simulink model "tiaoshi"  (R2014b)
settings: Solver=ode45  StartTime=0.0  StopTime=10.0  RelTol=1e-3
libraries: simulink x4, fuzblock x1
settings Model: Creator=Administrator  LastModifiedBy=Administrator

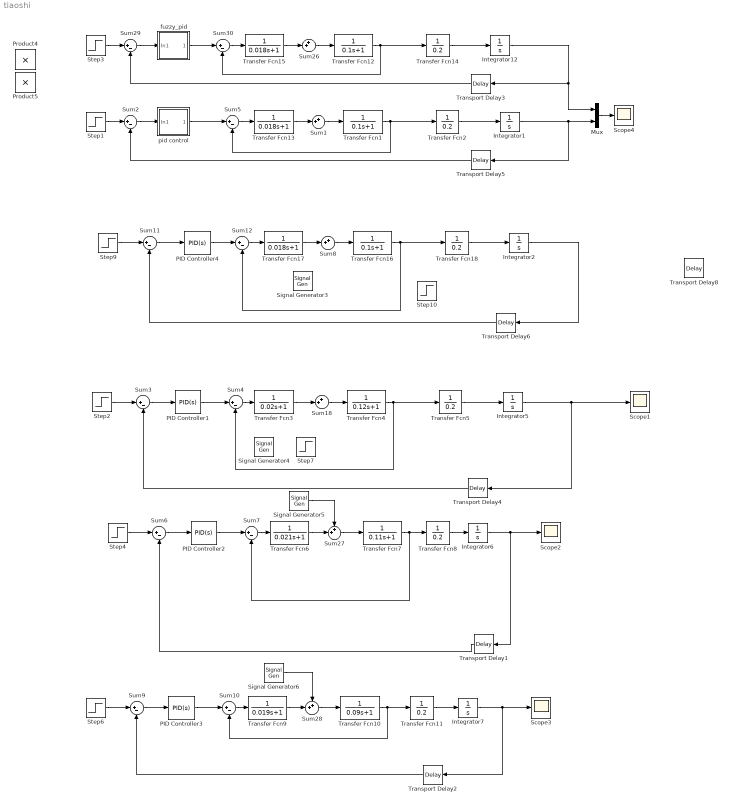
== system tiaoshi ==
  Integrator{1..2,5..7,12} (6 alike) : Integrator
  Mux : Mux  Inputs=2
  PID Controller1 : simulink/Continuous/PID Controller  Controller=PID  TimeDomain=Continuous-time  SampleTime=-1  IntegratorMethod=Forward Euler  FilterMethod=Forward Euler  Form=Parallel  P=4.34348893595362  I=0.409606906541511  D=0.190106280421876  N=113.521570556965  InitialConditionSource=internal  InitialConditionForIntegrator=0  InitialConditionForFilter=0  ExternalReset=none  LimitOutput=off  UpperSaturationLimit=inf  LowerSaturationLimit=-inf  LinearizeAsGain=on  AntiWindupMode=none  Kb=1  TrackingMode=off  Kt=1  PParamMin=[]  PParamMax=[]  IParamMin=[]  IParamMax=[]  DParamMin=[]  DParamMax=[]  NParamMin=[]  NParamMax=[]  KbParamMin=[]  KbParamMax=[]  KtParamMin=[]  KtParamMax=[]  POutMin=[]  POutMax=[]  IOutMin=[]  IOutMax=[]  DOutMin=[]  DOutMax=[]  NOutMin=[]  NOutMax=[]  KbOutMin=[]  KbOutMax=[]  KtOutMin=[]  KtOutMax=[]  IntegratorOutMin=[]  IntegratorOutMax=[]  FilterOutMin=[]  FilterOutMax=[]  SumOutMin=[]  SumOutMax=[]  SumI1OutMin=[]  SumI1OutMax=[]  SumI2OutMin=[]  SumI2OutMax=[]  SumI3OutMin=[]  SumI3OutMax=[]  SumDOutMin=[]  SumDOutMax=[]  SaturationOutMin=[]  SaturationOutMax=[]  IntegratorContinuousStateAttributes=''  IntegratorStateMustResolveToSignalObject=off  IntegratorRTWStateStorageClass=Auto  FilterContinuousStateAttributes=''  FilterStateMustResolveToSignalObject=off  FilterRTWStateStorageClass=Auto  DifferentiatorICPrevScaledInput=0  DifferentiatorOutMin=[]  DifferentiatorOutMax=[]  UseFilter=on
  PID Controller2 : simulink/Continuous/PID Controller  Controller=PID  TimeDomain=Continuous-time  SampleTime=-1  IntegratorMethod=Forward Euler  FilterMethod=Forward Euler  Form=Parallel  P=4.3714761921553  I=0.418612157121434  D=0.176716531069936  N=115.244644738995  InitialConditionSource=internal  InitialConditionForIntegrator=0  InitialConditionForFilter=0  ExternalReset=none  LimitOutput=off  UpperSaturationLimit=inf  LowerSaturationLimit=-inf  LinearizeAsGain=on  AntiWindupMode=none  Kb=1  TrackingMode=off  Kt=1  PParamMin=[]  PParamMax=[]  IParamMin=[]  IParamMax=[]  DParamMin=[]  DParamMax=[]  NParamMin=[]  NParamMax=[]  KbParamMin=[]  KbParamMax=[]  KtParamMin=[]  KtParamMax=[]  POutMin=[]  POutMax=[]  IOutMin=[]  IOutMax=[]  DOutMin=[]  DOutMax=[]  NOutMin=[]  NOutMax=[]  KbOutMin=[]  KbOutMax=[]  KtOutMin=[]  KtOutMax=[]  IntegratorOutMin=[]  IntegratorOutMax=[]  FilterOutMin=[]  FilterOutMax=[]  SumOutMin=[]  SumOutMax=[]  SumI1OutMin=[]  SumI1OutMax=[]  SumI2OutMin=[]  SumI2OutMax=[]  SumI3OutMin=[]  SumI3OutMax=[]  SumDOutMin=[]  SumDOutMax=[]  SaturationOutMin=[]  SaturationOutMax=[]  IntegratorContinuousStateAttributes=''  IntegratorStateMustResolveToSignalObject=off  IntegratorRTWStateStorageClass=Auto  FilterContinuousStateAttributes=''  FilterStateMustResolveToSignalObject=off  FilterRTWStateStorageClass=Auto  DifferentiatorICPrevScaledInput=0  DifferentiatorOutMin=[]  DifferentiatorOutMax=[]  UseFilter=on
  PID Controller3 : simulink/Continuous/PID Controller  Controller=PID  TimeDomain=Continuous-time  SampleTime=-1  IntegratorMethod=Forward Euler  FilterMethod=Forward Euler  Form=Parallel  P=4.54060551459518  I=0.450019772467081  D=0.137661903224342  N=119.172045893014  InitialConditionSource=internal  InitialConditionForIntegrator=0  InitialConditionForFilter=0  ExternalReset=none  LimitOutput=off  UpperSaturationLimit=inf  LowerSaturationLimit=-inf  LinearizeAsGain=on  AntiWindupMode=none  Kb=1  TrackingMode=off  Kt=1  PParamMin=[]  PParamMax=[]  IParamMin=[]  IParamMax=[]  DParamMin=[]  DParamMax=[]  NParamMin=[]  NParamMax=[]  KbParamMin=[]  KbParamMax=[]  KtParamMin=[]  KtParamMax=[]  POutMin=[]  POutMax=[]  IOutMin=[]  IOutMax=[]  DOutMin=[]  DOutMax=[]  NOutMin=[]  NOutMax=[]  KbOutMin=[]  KbOutMax=[]  KtOutMin=[]  KtOutMax=[]  IntegratorOutMin=[]  IntegratorOutMax=[]  FilterOutMin=[]  FilterOutMax=[]  SumOutMin=[]  SumOutMax=[]  SumI1OutMin=[]  SumI1OutMax=[]  SumI2OutMin=[]  SumI2OutMax=[]  SumI3OutMin=[]  SumI3OutMax=[]  SumDOutMin=[]  SumDOutMax=[]  SaturationOutMin=[]  SaturationOutMax=[]  IntegratorContinuousStateAttributes=''  IntegratorStateMustResolveToSignalObject=off  IntegratorRTWStateStorageClass=Auto  FilterContinuousStateAttributes=''  FilterStateMustResolveToSignalObject=off  FilterRTWStateStorageClass=Auto  DifferentiatorICPrevScaledInput=0  DifferentiatorOutMin=[]  DifferentiatorOutMax=[]  UseFilter=on
  PID Controller4 : simulink/Continuous/PID Controller  Controller=PID  TimeDomain=Continuous-time  SampleTime=-1  IntegratorMethod=Forward Euler  FilterMethod=Forward Euler  Form=Parallel  P=7.09807299066698  I=1.09867748930147  D=0.315560684469702  N=2035.68968381362  InitialConditionSource=internal  InitialConditionForIntegrator=0  InitialConditionForFilter=0  ExternalReset=none  LimitOutput=off  UpperSaturationLimit=inf  LowerSaturationLimit=-inf  LinearizeAsGain=on  AntiWindupMode=none  Kb=1  TrackingMode=off  Kt=1  PParamMin=[]  PParamMax=[]  IParamMin=[]  IParamMax=[]  DParamMin=[]  DParamMax=[]  NParamMin=[]  NParamMax=[]  KbParamMin=[]  KbParamMax=[]  KtParamMin=[]  KtParamMax=[]  POutMin=[]  POutMax=[]  IOutMin=[]  IOutMax=[]  DOutMin=[]  DOutMax=[]  NOutMin=[]  NOutMax=[]  KbOutMin=[]  KbOutMax=[]  KtOutMin=[]  KtOutMax=[]  IntegratorOutMin=[]  IntegratorOutMax=[]  FilterOutMin=[]  FilterOutMax=[]  SumOutMin=[]  SumOutMax=[]  SumI1OutMin=[]  SumI1OutMax=[]  SumI2OutMin=[]  SumI2OutMax=[]  SumI3OutMin=[]  SumI3OutMax=[]  SumDOutMin=[]  SumDOutMax=[]  SaturationOutMin=[]  SaturationOutMax=[]  IntegratorContinuousStateAttributes=''  IntegratorStateMustResolveToSignalObject=off  IntegratorRTWStateStorageClass=Auto  FilterContinuousStateAttributes=''  FilterStateMustResolveToSignalObject=off  FilterRTWStateStorageClass=Auto  DifferentiatorICPrevScaledInput=0  DifferentiatorOutMin=[]  DifferentiatorOutMax=[]  UseFilter=on
  Product4 : Product  RndMeth=Zero
  Product5 : Product  RndMeth=Zero
  Scope{1..4} (4 alike) : Scope
      Scope1 settings: SaveName=dianji2
      Scope2 settings: SaveName=dianji3
      Scope3 settings: SaveName=dianji4
      Scope4 settings: SaveName=dianjix
  Signal Generator{3..6} (4 alike) : SignalGenerator  WaveForm=random  Amplitude=10  Frequency=2
  Step{1..3,9} (4 alike) : Step  After=50  SampleTime=0
  Step10 : Step  Time=5  After=-1  SampleTime=0
  Step4 : Step  SampleTime=0
  Step6 : Step  SampleTime=0
  Step7 : Step  Time=5  After=-1  SampleTime=0
  Sum{1,8,18,26..28} (6 alike) : Sum  Inputs=++|
  Sum{2..7,9..12,29..30} (12 alike) : Sum  Inputs=|+-
  Transfer Fcn1 : TransferFcn  Denominator=[0.1 1]
  Transfer Fcn10 : TransferFcn  Denominator=[0.09 1]
  Transfer Fcn{2,5,8,11,14,18} (6 alike) : TransferFcn  Denominator=[0.2]
  Transfer Fcn12 : TransferFcn  Denominator=[0.1 1]
  Transfer Fcn13 : TransferFcn  Denominator=[0.018 1]
  Transfer Fcn15 : TransferFcn  Denominator=[0.018 1]
  Transfer Fcn16 : TransferFcn  Denominator=[0.1 1]
  Transfer Fcn17 : TransferFcn  Denominator=[0.018 1]
  Transfer Fcn3 : TransferFcn  Denominator=[0.02 1]
  Transfer Fcn4 : TransferFcn  Denominator=[0.12 1]
  Transfer Fcn6 : TransferFcn  Denominator=[0.021 1]
  Transfer Fcn7 : TransferFcn  Denominator=[0.11 1]
  Transfer Fcn9 : TransferFcn  Denominator=[0.019 1]
  Transport Delay1 : TransportDelay  DelayTime=0.02
  Transport Delay2 : TransportDelay  DelayTime=0.02
  Transport Delay{3,5..6,8} (4 alike) : TransportDelay  DelayTime=0.004
  Transport Delay4 : TransportDelay  DelayTime=0.02
  fuzzy_pid : Subsystem
  pid control : Subsystem
  wires:
  Step2/1 -> Sum3/1
  Sum3/1 -> PID Controller1/1
  Transfer Fcn4/1 -> Sum4/2, Transfer Fcn5/1
  Sum4/1 -> Transfer Fcn3/1
  PID Controller1/1 -> Sum4/1
  Transfer Fcn5/1 -> Integrator5/1
  Step4/1 -> Sum6/1
  Sum6/1 -> PID Controller2/1
  Transfer Fcn7/1 -> Transfer Fcn8/1, Sum7/2
  Sum7/1 -> Transfer Fcn6/1
  PID Controller2/1 -> Sum7/1
  Transfer Fcn8/1 -> Integrator6/1
  Step6/1 -> Sum9/1
  Sum9/1 -> PID Controller3/1
  Transfer Fcn10/1 -> Transfer Fcn11/1, Sum10/2
  Sum10/1 -> Transfer Fcn9/1
  PID Controller3/1 -> Sum10/1
  Transfer Fcn11/1 -> Integrator7/1
  Integrator6/1 -> Scope2/1, Transport Delay1/1
  Integrator7/1 -> Transport Delay2/1, Scope3/1
  Transfer Fcn3/1 -> Sum18/2
  Sum18/1 -> Transfer Fcn4/1
  Integrator5/1 -> Scope1/1, Transport Delay4/1
  Transport Delay4/1 -> Sum3/2
  Transport Delay1/1 -> Sum6/2
  Transport Delay2/1 -> Sum9/2
  Signal Generator5/1 -> Sum27/1
  Transfer Fcn6/1 -> Sum27/2
  Sum27/1 -> Transfer Fcn7/1
  Transfer Fcn9/1 -> Sum28/2
  Sum28/1 -> Transfer Fcn10/1
  Signal Generator6/1 -> Sum28/1
  Step3/1 -> Sum29/1
  Sum29/1 -> fuzzy_pid/1(In1)
  Transfer Fcn12/1 -> Sum30/2, Transfer Fcn14/1
  Sum30/1 -> Transfer Fcn15/1
  Transfer Fcn14/1 -> Integrator12/1
  Sum26/1 -> Transfer Fcn12/1
  Integrator12/1 -> Mux/1, Transport Delay3/1
  Transport Delay3/1 -> Sum29/2
  Transfer Fcn15/1 -> Sum26/2
  fuzzy_pid/1(Out1) -> Sum30/1
  Step1/1 -> Sum2/1
  Transfer Fcn1/1 -> Sum5/2, Transfer Fcn2/1
  Sum5/1 -> Transfer Fcn13/1
  Transfer Fcn2/1 -> Integrator1/1
  Sum1/1 -> Transfer Fcn1/1
  Integrator1/1 -> Mux/2, Transport Delay5/1
  Transport Delay5/1 -> Sum2/2
  Transfer Fcn13/1 -> Sum1/2
  pid control/1(Out1) -> Sum5/1
  Mux/1 -> Scope4/1
  Step9/1 -> Sum11/1
  Sum11/1 -> PID Controller4/1
  Transfer Fcn16/1 -> Sum12/2, Transfer Fcn18/1
  Sum12/1 -> Transfer Fcn17/1
  Transfer Fcn18/1 -> Integrator2/1
  Sum8/1 -> Transfer Fcn16/1
  Integrator2/1 -> Transport Delay6/1
  Transport Delay6/1 -> Sum11/2
  Transfer Fcn17/1 -> Sum8/2
  PID Controller4/1 -> Sum12/1
  Sum2/1 -> pid control/1(In1)

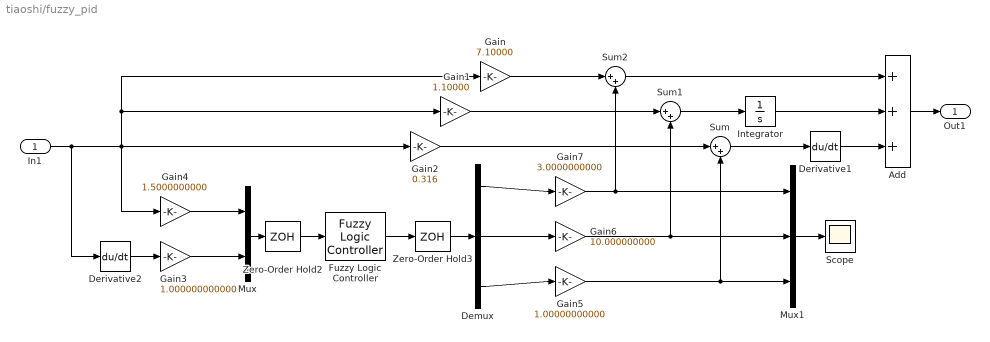
== system tiaoshi/fuzzy_pid ==
  In1 : Inport
  Add : Sum  Inputs=+++
  Demux : Demux  Outputs=3
  Derivative1 : Derivative
  Derivative2 : Derivative
  Fuzzy Logic Controller : fuzblock/Fuzzy Logic  Controller  fis=fuzzy_1
  Gain : Gain  Gain=7.10000
  Gain1 : Gain  Gain=1.10000
  Gain2 : Gain  Gain=0.316
  Gain3 : Gain  Gain=1.000000000000
  Gain4 : Gain  Gain=1.5000000000
  Gain5 : Gain  Gain=1.00000000000
  Gain6 : Gain  Gain=10.000000000
  Gain7 : Gain  Gain=3.0000000000
  Integrator : Integrator
  Mux : Mux  Inputs=2
  Mux1 : Mux  Inputs=3
  Scope : Scope
  Sum : Sum  Inputs=|++
  Sum1 : Sum  Inputs=|++
  Sum2 : Sum  Inputs=|++
  Zero-Order Hold2 : ZeroOrderHold  SampleTime=0.01
  Zero-Order Hold3 : ZeroOrderHold  SampleTime=0.01
  Out1 : Outport
  wires:
  Derivative1/1 -> Add/3
  Integrator/1 -> Add/2
  Add/1 -> Out1/1
  Gain/1 -> Sum2/1
  Gain1/1 -> Sum1/1
  Gain2/1 -> Sum/1
  Mux/1 -> Zero-Order Hold2/1
  Fuzzy Logic Controller/1 -> Zero-Order Hold3/1
  Mux1/1 -> Scope/1
  Zero-Order Hold2/1 -> Fuzzy Logic Controller/1
  Zero-Order Hold3/1 -> Demux/1
  Gain7/1 -> Sum2/2, Mux1/1
  Gain6/1 -> Mux1/2, Sum1/2
  Gain5/1 -> Sum/2, Mux1/3
  Gain4/1 -> Mux/1
  Gain3/1 -> Mux/2
  Derivative2/1 -> Gain3/1
  In1/1 -> Derivative2/1, Gain1/1, Gain/1, Gain2/1, Gain4/1
  Demux/1 -> Gain7/1
  Demux/2 -> Gain6/1
  Demux/3 -> Gain5/1
  Sum2/1 -> Add/1
  Sum1/1 -> Integrator/1
  Sum/1 -> Derivative1/1

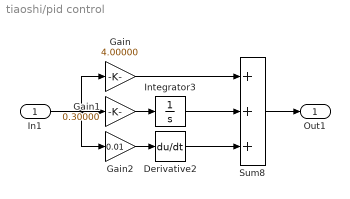
== system tiaoshi/pid control ==
  In1 : Inport
  Derivative2 : Derivative
  Gain : Gain  Gain=4.00000
  Gain1 : Gain  Gain=0.30000
  Gain2 : Gain  Gain=0.01
  Integrator3 : Integrator
  Sum8 : Sum  Inputs=+++
  Out1 : Outport
  wires:
  Gain1/1 -> Integrator3/1
  Gain/1 -> Sum8/1
  Derivative2/1 -> Sum8/3
  Gain2/1 -> Derivative2/1
  Sum8/1 -> Out1/1
  In1/1 -> Gain2/1, Gain/1, Gain1/1
  Integrator3/1 -> Sum8/2
